simulink model "EVdemo_6"  (R2013b)
settings: Solver=FixedStepDiscrete  SolverMode=SingleTasking  StartTime=0.0  StopTime=650  FixedStep=4e-5  MaxStep=1e-5  RelTol=1e-3
InitFcn:
  | %EV_Param_Update
  | % update the number of strings (discretized)
  | numStrings = round(Opti_numStrings);
  | %disp(['Number of strings: ' num2str(numStrings)])
  | % update the effective capacity based on the number of strings
  | EV_Param.Battery_Det.Rated_Capacity = 28.5*numStrings; %A*hr
  | EV_Param.Battery_Det.DP = 1.5*fliplr([1500 1500 1600 1450 1325 1125 925 675 425 175 ])./8*EV_Param.Battery_Det.Rated_Capacity; % 8 comes from the 8Ahr rated batter data used (normalize and rescale to the rated capacity
  | EV_Param.Battery_Det.CP = fliplr([25 100 200 250 375 550 750 950 1125 1150])./8*EV_Param.Battery_Det.Rated_Capacity;
  | 
  | % update the number of cells in a string (discretized)
  | numSeriesCells = round(Opti_numSeriesCells);
  | %disp(['Number of cells in a string: ' num2str(numSeriesCells)])
  | % update the nominal string volage and charge deficit
  | EV_Param.Battery_Det.Nominal_Voltage = numSeriesCells*cellVolts;
  | BatteryParams(1).Qe_init = 0;%EV_Param.Battery_Det.Rated_Capacity*(1-EV_Param.Battery_Det.Initial_SOC/100); %Ampere*hours
  | 
  | % update the total number of cells, battery pack mass and total vehicle
  | % mass
  | total_cells = numSeriesCells*numStrings;
  | %disp(['Total Number of cells: ' num2str(total_cells)])
  | EV_Param.BatteryMass = BatteryParams(1).cell_mass*total_cells;
  | %disp(['Total Battery Pack Mass: ' num2str(EV_Param.BatteryMass)])
  | EV_Param.Vehicle.Mass = 1300+EV_Param.BatteryMass;
  | 
  | % update the driveline gear ratio
  | EV_Param.Vehicle.Engine_Vehicle_Gear_Ratio = Opti_Vehicle_Gear_Ratio;
  | %disp(['Driveline gear ratio: ' num2str(Opti_Vehicle_Gear_Ratio)])
StartFcn:
  | %tic;
StopFcn:
  | %toc;
  | %disp([Final SOC: ' num2str(SOC_final)])
  | %disp([Final Vehicle Error: ' num2str(normed_SQE_final)])
model workspace (MAT data in the model file):
  MCOS : class17 (value not decoded)
  MCOS : class17 (value not decoded)
values from neighbouring files (symbols this model uses):
  Drive_Cycle_Num = 8    [startDemo.m]
undefined symbols (not defined in the file or in its folder): Acc_Cmd, BatteryParams, Brake_Set, cell_area, ctrlConst, current_phase_a, Dec_Cmd, direct_current, DiscIntNeverNeededParam, electromagnetic_torque, HEV_Param, Ion, Kt_Temps, Lithium, Mech_Power_kW, Opti_numSeriesCells, Opti_numStrings, Opti_Vehicle_Gear_Ratio, paramVelocityI, paramVelocityP, paramVelocityPICurrentSat, pmsm, quadrature_current, RLoadLoss, rotor_velocity, sigbuilder_block, Ts, Veh_Spd_Ref
libraries: fl_lib x306, nesl_utility x100, LeadAcidBattery_lib x60, simulink x23, powerlib x16, sdl_lib x7, elec_lib x4, electricdrivelib x2, checkpacklib x2, CustomDriveline_lib x2, LiBatteryBlocks x1, Capacitors_lib x1
(part 4 of 7)

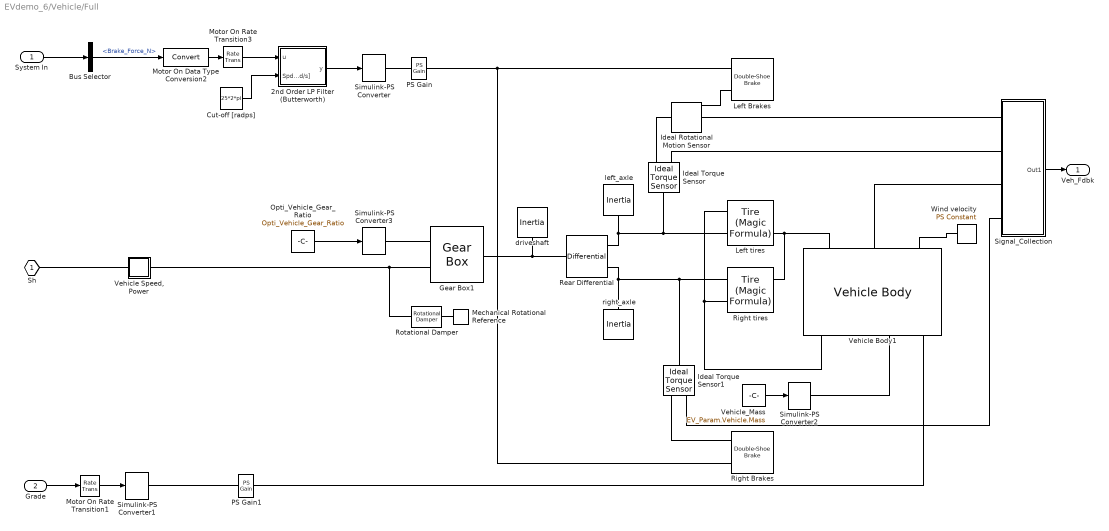
== system EVdemo_6/Vehicle/Full ==
  System In : Inport
  Grade : Inport  Port=2
  2nd Order LP Filter (Butterworth) : Subsystem  mask{DT=1e-3}
      mask prompts: DT "Sampe Time"
      mask Display:
      | plot([0 0],[0 1]);
      | plot([0 1],[0 0]);
      | plot([0 .5 .75 1],[1 1 .7071 .01]);
  Bus Selector : BusSelector  OutputSignals=Brake_Force_N
  Cut-off [radps] : Constant  Value=25*2*pi  OutDataTypeStr=single  SampleTime=-1
  Gear Box1 : CustomDriveline_lib/Gear Box  ratio_min=1  t_in_Log=off  t_out_Log=off  LocalVarNames=|t_in|t_out  LocalVarDescs=|t_in|t_out  LocalVarLogging=[0 0]
  Ideal Rotational Motion Sensor : fl_lib/Mechanical/Mechanical Sensors/Ideal Rotational Motion Sensor  offset=0 rad  w_Log=off  t_Log=off  phi_Log=off  LocalVarNames=|w|t|phi  LocalVarDescs=|w|t|phi  LocalVarLogging=[0 0 0]
  Ideal Torque Sensor : fl_lib/Mechanical/Mechanical Sensors/Ideal Torque Sensor  w_Log=off  t_Log=off  LocalVarNames=|w|t  LocalVarDescs=|w|t  LocalVarLogging=[0 0]
  Ideal Torque Sensor1 : fl_lib/Mechanical/Mechanical Sensors/Ideal Torque Sensor  w_Log=off  t_Log=off  LocalVarNames=|w|t  LocalVarDescs=|w|t  LocalVarLogging=[0 0]
  Left Brakes : sdl_lib/Brakes & Detents/Rotational/Double-Shoe Brake  r_drum=150 mm  r_act=125 mm  r_pin=125 mm  theta_pin=15 deg  theta_0=5 deg  theta_shoe=120 deg  mu_visc=.01 N*m/(rad/s)  mu=0.3  w_thr=0.1 rad/s  w_shaft_Log=off  t_shaft_Log=off  LocalVarNames=|w_shaft|t_shaft  LocalVarDescs=|Rotational velocity of the shaft|Braking torque on the shaft  LocalVarLogging=[0 0]  mask(Double-Shoe Brake){}
      mask Display:
      | % This is a new mask on top of the base mask.
      | % Use "View base mask" link below to see the base mask.
      | image('brakes.jpg')
  Left tires : sdl_lib/Tires & Vehicles/Tire (Magic Formula)  parameterization=1  F_z1=EV_Param.Vehicle.Tire.Rated_Vertical_Load N  F_x1=EV_Param.Vehicle.Tire.Rated_Peak_Long_Force N  kappa1=EV_Param.Vehicle.Tire.Slip_At_Peak_Force  B_m=10  C_m=1.9  D_m=1  E_m=0.97  fz0=4e+3 N  p_Cx=1.685  p_Dx=[ 1.21 -0.037 ]  p_Ex=[ 0.344 0.095 -0.02 0 ]  p_Kx=[ 21.51 -0.163 0.245 ]  p_Hx=[ -0.002 0.002 ]  p_Vx=[ 0 0 ]  v_tr_thr=0.1 m/s  r_e=EV_Param.Vehicle.Tire_Radius m  model_compliance=0  stiffness=1e+6 N/m  damping=1000 N/(m/s)  model_inertia=1  inertia=1e-2 kg*m^2  initial_velocity=0 rpm  model_resistance=1  resistance_model=2  coeff=0.015  p_tire=250e3 Pa  alpha=-0.003  beta=0.97  coeff_a=84e-4  coeff_b=6.2e-4 s/m  coeff_c=1.6e-4 s^2/m^2  v_thr=1e-2 m/s  LocalVarLogging=[]
  Mechanical Rotational Reference : fl_lib/Mechanical/Rotational Elements/Mechanical Rotational Reference  t_Log=off  LocalVarNames=|t  LocalVarDescs=|t  LocalVarLogging=0
  Motor On Data Type Conversion2 : DataTypeConversion
  Motor On Rate Transition1 : RateTransition  Deterministic=off
  Motor On Rate Transition3 : RateTransition  Deterministic=off
  Opti_Vehicle_Gear_Ratio : Constant  Value=Opti_Vehicle_Gear_Ratio  OutDataTypeStr=double  SampleTime=-1
  PS Gain : fl_lib/Physical Signals/Functions/PS Gain  gain=1  LocalVarLogging=[]
  PS Gain1 : fl_lib/Physical Signals/Functions/PS Gain  gain=1  LocalVarLogging=[]
  Rear Differential : sdl_lib/Gears/Differential  driveshaft_location=2  cd_ratio=1  friction_model=1  efficiency=[ 0.85 0.92 ]  mu_visc=[ 0 0 ] N*m/(rad/s)  w_thr=[ 0.01 0.01 ] rad/s  LocalVarLogging=[]
  Right Brakes : sdl_lib/Brakes & Detents/Rotational/Double-Shoe Brake  r_drum=150 mm  r_act=125 mm  r_pin=125 mm  theta_pin=15 deg  theta_0=5 deg  theta_shoe=120 deg  mu_visc=.01 N*m/(rad/s)  mu=0.3  w_thr=0.1 rad/s  w_shaft_Log=off  t_shaft_Log=off  LocalVarNames=|w_shaft|t_shaft  LocalVarDescs=|Rotational velocity of the shaft|Braking torque on the shaft  LocalVarLogging=[0 0]  mask(Double-Shoe Brake){}
      mask Display:
      | % This is a new mask on top of the base mask.
      | % Use "View base mask" link below to see the base mask.
      | image('brakes.jpg')
  Right tires : sdl_lib/Tires & Vehicles/Tire (Magic Formula)  parameterization=1  F_z1=EV_Param.Vehicle.Tire.Rated_Vertical_Load N  F_x1=EV_Param.Vehicle.Tire.Rated_Peak_Long_Force N  kappa1=EV_Param.Vehicle.Tire.Slip_At_Peak_Force  B_m=10  C_m=1.9  D_m=1  E_m=0.97  fz0=4e+3 N  p_Cx=1.685  p_Dx=[ 1.21 -0.037 ]  p_Ex=[ 0.344 0.095 -0.02 0 ]  p_Kx=[ 21.51 -0.163 0.245 ]  p_Hx=[ -0.002 0.002 ]  p_Vx=[ 0 0 ]  v_tr_thr=0.1 m/s  r_e=EV_Param.Vehicle.Tire_Radius m  model_compliance=0  stiffness=1e+6 N/m  damping=1000 N/(m/s)  model_inertia=1  inertia=1e-2 kg*m^2  initial_velocity=0 rpm  model_resistance=1  resistance_model=2  coeff=0.015  p_tire=250e3 Pa  alpha=-0.003  beta=0.97  coeff_a=84e-4  coeff_b=6.2e-4 s/m  coeff_c=1.6e-4 s^2/m^2  v_thr=1e-2 m/s  LocalVarLogging=[]
  Rotational Damper : fl_lib/Mechanical/Rotational Elements/Rotational Damper  D=EV_Param.Vehicle.Trans.Friction N*m/(rad/s)  t_Log=off  w_Log=off  LocalVarNames=|t|w  LocalVarDescs=|t|w  LocalVarLogging=[0 0]
  Signal_Collection : Subsystem
  Simulink-PS Converter : nesl_utility/Simulink-PS Converter  PhysicalDomain=network_engine_domain  SubClassName=ps_input  LeftPortType=input  RightPortType=output  PseudoPeriodic=off  Frequencies=[]  NoiseDistribution=none  NoiseParameters=[]  Unit=N  AffineConversion=off  InputFiltering=off  SimscapeFilterOrder=1  InputFilterTimeConstant=0.001  UdotUserProvided=1
  Simulink-PS Converter1 : nesl_utility/Simulink-PS Converter  PhysicalDomain=network_engine_domain  SubClassName=ps_input  LeftPortType=input  RightPortType=output  PseudoPeriodic=off  Frequencies=[]  NoiseDistribution=none  NoiseParameters=[]  Unit=rad  AffineConversion=off  InputFiltering=off  SimscapeFilterOrder=1  InputFilterTimeConstant=0.001  UdotUserProvided=1
  Simulink-PS Converter2 : nesl_utility/Simulink-PS Converter  PhysicalDomain=network_engine_domain  SubClassName=ps_input  LeftPortType=input  RightPortType=output  PseudoPeriodic=off  Frequencies=[]  NoiseDistribution=none  NoiseParameters=[]  Unit=kg  AffineConversion=off  InputFiltering=off  SimscapeFilterOrder=1  InputFilterTimeConstant=0.001  UdotUserProvided=1
  Simulink-PS Converter3 : nesl_utility/Simulink-PS Converter  PhysicalDomain=network_engine_domain  SubClassName=ps_input  LeftPortType=input  RightPortType=output  PseudoPeriodic=off  Frequencies=[]  NoiseDistribution=none  NoiseParameters=[]  Unit=1  AffineConversion=off  InputFiltering=off  SimscapeFilterOrder=1  InputFilterTimeConstant=0.001  UdotUserProvided=1
  "Vehicle Speed, Power" : Subsystem
      mask Display: disp('S')
  Vehicle Body1 : CustomDriveline_lib/Vehicle Body  n_w=2  x_f=EV_Param.Vehicle.Distance_CG_FrontAxle m  x_r=EV_Param.Vehicle.Distance_CG_RearAxle m  y_c=EV_Param.Vehicle.Distance_CG_Ground m  area=EV_Param.Vehicle.Frontal_Area m^2  Cd=EV_Param.Vehicle.Aero_Drag_Coeff  v0=0 m/s  g=9.81 m/s^2  rho=1.18 kg/m^3  mass_min=1e-3 kg  LocalVarLogging=[]
  Vehicle_Mass : Constant  Value=EV_Param.Vehicle.Mass  OutDataTypeStr=double  SampleTime=-1
  Wind velocity : fl_lib/Physical Signals/Sources/PS Constant  constant=0  LocalVarLogging=[]
  driveshaft : fl_lib/Mechanical/Rotational Elements/Inertia  inertia=EV_Param.Vehicle.Trans.Inertia kg*m^2  initial_velocity=0 rad/s  t_Log=off  LocalVarNames=|t  LocalVarDescs=|t  LocalVarLogging=0
  left_axle : fl_lib/Mechanical/Rotational Elements/Inertia  inertia=EV_Param.Vehicle.Wheel_Inertia*2 kg*m^2  initial_velocity=0 rad/s  t_Log=off  LocalVarNames=|t  LocalVarDescs=|t  LocalVarLogging=0
  right_axle : fl_lib/Mechanical/Rotational Elements/Inertia  inertia=EV_Param.Vehicle.Wheel_Inertia*2 kg*m^2  initial_velocity=0 rad/s  t_Log=off  LocalVarNames=|t  LocalVarDescs=|t  LocalVarLogging=0
  Sh : PMIOPort  Port=1  Side=Left
  Veh_Fdbk : Outport
  wires:
  Bus Selector/1 -> Motor On Data Type Conversion2/1  "<Brake_Force_N>"
  System In/1 -> Bus Selector/1
  Motor On Data Type Conversion2/1 -> Motor On Rate Transition3/1
  Motor On Rate Transition1/1 -> Simulink-PS Converter1/1
  Grade/1 -> Motor On Rate Transition1/1
  Signal_Collection/1(Out1) -> Veh_Fdbk/1
  Motor On Rate Transition3/1 -> 2nd Order LP Filter (Butterworth)/1(u)
  Cut-off [radps]/1 -> 2nd Order LP Filter (Butterworth)/2(Spd_Err_Filt_BW [rad/s])
  2nd Order LP Filter (Butterworth)/1(y) -> Simulink-PS Converter/1
  Vehicle_Mass/1 -> Simulink-PS Converter2/1
  Opti_Vehicle_Gear_Ratio/1 -> Simulink-PS Converter3/1
  connections:
  Right tires/RConn2 -- Vehicle Body1/LConn1 -- Left tires/RConn2
  Right tires/LConn1 -- Left tires/LConn1 -- Vehicle Body1/RConn1
  PS Gain1/RConn1 -- Vehicle Body1/RConn4
  Wind velocity/RConn1 -- Vehicle Body1/LConn3
  Rear Differential/RConn2 -- Left tires/LConn2 -- Ideal Torque Sensor/LConn1 -- left_axle/LConn1
  Right tires/LConn2 -- Ideal Torque Sensor1/LConn1 -- Rear Differential/RConn1 -- right_axle/LConn1
  Rear Differential/LConn1 -- Gear Box1/RConn1 -- driveshaft/LConn1
  "Vehicle Speed, Power"/RConn1 -- Gear Box1/LConn2 -- Rotational Damper/LConn1
  Rotational Damper/RConn1 -- Mechanical Rotational Reference/LConn1
  Sh/RConn1 -- "Vehicle Speed, Power"/LConn1
  PS Gain/RConn1 -- Right Brakes/LConn1 -- Left Brakes/LConn1
  Simulink-PS Converter/RConn1 -- PS Gain/LConn1
  Simulink-PS Converter1/RConn1 -- PS Gain1/LConn1
  Ideal Torque Sensor/RConn1 -- Ideal Rotational Motion Sensor/LConn1
  Ideal Torque Sensor1/RConn1 -- Right Brakes/LConn2
  Ideal Rotational Motion Sensor/RConn1 -- Left Brakes/LConn2
  Ideal Rotational Motion Sensor/RConn2 -- Signal_Collection/LConn1
  Ideal Torque Sensor/RConn2 -- Signal_Collection/LConn2
  Vehicle Body1/LConn2 -- Signal_Collection/LConn3
  Ideal Torque Sensor1/RConn2 -- Signal_Collection/LConn4
  Simulink-PS Converter2/RConn1 -- Vehicle Body1/RConn3
  Simulink-PS Converter3/RConn1 -- Gear Box1/LConn1

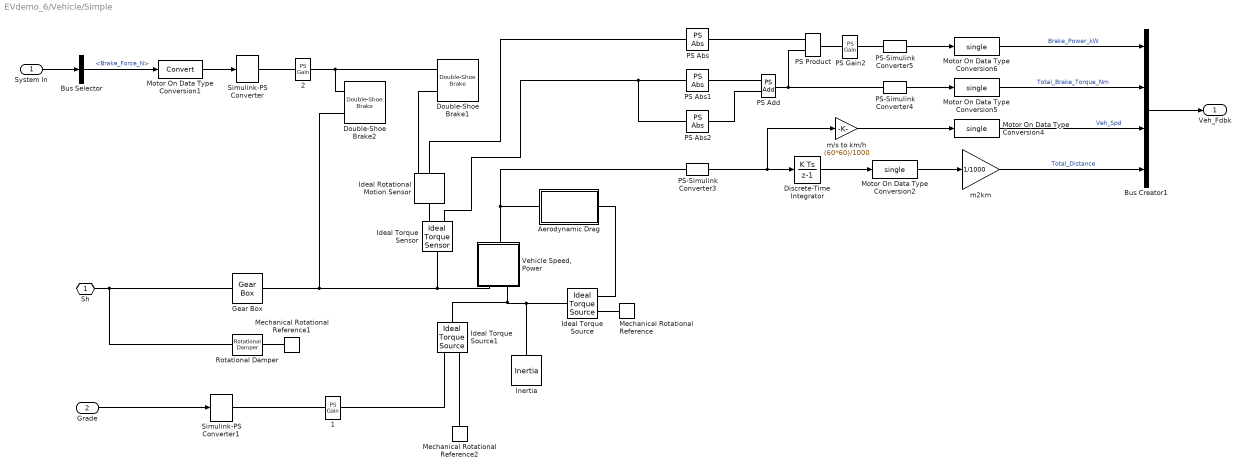
== system EVdemo_6/Vehicle/Simple ==
  System In : Inport
  Grade : Inport  Port=2
  1 : fl_lib/Physical Signals/Functions/PS Gain  gain=0  LocalVarLogging=[]
  2 : fl_lib/Physical Signals/Functions/PS Gain  gain=1  LocalVarLogging=[]
  Aerodynamic Drag : Subsystem
  Bus Creator1 : BusCreator
  Bus Selector : BusSelector  OutputSignals=Brake_Force_N
  Discrete-Time Integrator : DiscreteIntegrator  SampleTime=-1  ICPrevOutput=DiscIntNeverNeededParam  ICPrevScaledInput=DiscIntNeverNeededParam
  Double-Shoe Brake1 : sdl_lib/Brakes & Detents/Rotational/Double-Shoe Brake  r_drum=150 mm  r_act=125 mm  r_pin=125 mm  theta_pin=15 deg  theta_0=5 deg  theta_shoe=120 deg  mu_visc=.01 N*m/(rad/s)  mu=0.3  w_thr=0.1 rad/s  w_shaft_Log=off  t_shaft_Log=off  LocalVarNames=|w_shaft|t_shaft  LocalVarDescs=|Rotational velocity of the shaft|Braking torque on the shaft  LocalVarLogging=[0 0]
  Double-Shoe Brake2 : sdl_lib/Brakes & Detents/Rotational/Double-Shoe Brake  r_drum=150 mm  r_act=125 mm  r_pin=125 mm  theta_pin=15 deg  theta_0=5 deg  theta_shoe=120 deg  mu_visc=.01 N*m/(rad/s)  mu=0.3  w_thr=0.1 rad/s  w_shaft_Log=off  t_shaft_Log=off  LocalVarNames=|w_shaft|t_shaft  LocalVarDescs=|Rotational velocity of the shaft|Braking torque on the shaft  LocalVarLogging=[0 0]
  Gear Box : fl_lib/Mechanical/Mechanisms/Gear Box  ratio=gear_ratio  t_in_Log=off  t_out_Log=off  LocalVarNames=|t_in|t_out  LocalVarDescs=|t_in|t_out  LocalVarLogging=[0 0]
  Ideal Rotational Motion Sensor : fl_lib/Mechanical/Mechanical Sensors/Ideal Rotational Motion Sensor  offset=0 rad  w_Log=off  t_Log=off  phi_Log=off  LocalVarNames=|w|t|phi  LocalVarDescs=|w|t|phi  LocalVarLogging=[0 0 0]
  Ideal Torque Sensor : fl_lib/Mechanical/Mechanical Sensors/Ideal Torque Sensor  w_Log=off  t_Log=off  LocalVarNames=|w|t  LocalVarDescs=|w|t  LocalVarLogging=[0 0]
  Ideal Torque Source : fl_lib/Mechanical/Mechanical Sources/Ideal Torque Source  w_Log=off  t_Log=off  LocalVarNames=|w|t  LocalVarDescs=|w|t  LocalVarLogging=[0 0]
  Ideal Torque Source1 : fl_lib/Mechanical/Mechanical Sources/Ideal Torque Source  w_Log=off  t_Log=off  LocalVarNames=|w|t  LocalVarDescs=|w|t  LocalVarLogging=[0 0]
  Inertia : fl_lib/Mechanical/Rotational Elements/Inertia  inertia=4*wheel_inertia+mass*radius*radius kg*m^2  initial_velocity=0 rad/s  t_Log=off  LocalVarNames=|t  LocalVarDescs=|t  LocalVarLogging=0
  Mechanical Rotational Reference : fl_lib/Mechanical/Rotational Elements/Mechanical Rotational Reference  t_Log=off  LocalVarNames=|t  LocalVarDescs=|t  LocalVarLogging=0
  Mechanical Rotational Reference1 : fl_lib/Mechanical/Rotational Elements/Mechanical Rotational Reference  t_Log=off  LocalVarNames=|t  LocalVarDescs=|t  LocalVarLogging=0
  Mechanical Rotational Reference2 : fl_lib/Mechanical/Rotational Elements/Mechanical Rotational Reference  t_Log=off  LocalVarNames=|t  LocalVarDescs=|t  LocalVarLogging=0
  Motor On Data Type Conversion1 : DataTypeConversion
  Motor On Data Type Conversion{2,4..6} (4 alike) : DataTypeConversion  OutDataTypeStr=single
  PS Abs : fl_lib/Physical Signals/Nonlinear Operators/PS Abs  LocalVarLogging=[]
  PS Abs1 : fl_lib/Physical Signals/Nonlinear Operators/PS Abs  LocalVarLogging=[]
  PS Abs2 : fl_lib/Physical Signals/Nonlinear Operators/PS Abs  LocalVarLogging=[]
  PS Add : fl_lib/Physical Signals/Functions/PS Add  LocalVarLogging=[]
  PS Gain2 : fl_lib/Physical Signals/Functions/PS Gain  gain=1e-3  LocalVarLogging=[]
  PS Product : fl_lib/Physical Signals/Functions/PS Product  LocalVarLogging=[]
  PS-Simulink Converter3 : nesl_utility/PS-Simulink Converter  PhysicalDomain=network_engine_domain  SubClassName=ps_output  LeftPortType=input  RightPortType=output  PseudoPeriodic=off  Frequencies=[]  Unit=m/s  AffineConversion=off
  PS-Simulink Converter4 : nesl_utility/PS-Simulink Converter  PhysicalDomain=network_engine_domain  SubClassName=ps_output  LeftPortType=input  RightPortType=output  PseudoPeriodic=off  Frequencies=[]  Unit=m/s  AffineConversion=off
  PS-Simulink Converter5 : nesl_utility/PS-Simulink Converter  PhysicalDomain=network_engine_domain  SubClassName=ps_output  LeftPortType=input  RightPortType=output  PseudoPeriodic=off  Frequencies=[]  Unit=m/s  AffineConversion=off
  Rotational Damper : fl_lib/Mechanical/Rotational Elements/Rotational Damper  D=EV_Param.Vehicle.Trans.Friction N*m/(rad/s)  t_Log=off  w_Log=off  LocalVarNames=|t|w  LocalVarDescs=|t|w  LocalVarLogging=[0 0]
  Simulink-PS Converter : nesl_utility/Simulink-PS Converter  PhysicalDomain=network_engine_domain  SubClassName=ps_input  LeftPortType=input  RightPortType=output  PseudoPeriodic=off  Frequencies=[]  NoiseDistribution=none  NoiseParameters=[]  Unit=N  AffineConversion=off  InputFiltering=off  SimscapeFilterOrder=1  InputFilterTimeConstant=0.001  UdotUserProvided=1
  Simulink-PS Converter1 : nesl_utility/Simulink-PS Converter  PhysicalDomain=network_engine_domain  SubClassName=ps_input  LeftPortType=input  RightPortType=output  PseudoPeriodic=off  Frequencies=[]  NoiseDistribution=none  NoiseParameters=[]  Unit=N  AffineConversion=off  InputFiltering=off  SimscapeFilterOrder=1  InputFilterTimeConstant=0.001  UdotUserProvided=1
  "Vehicle Speed, Power" : Subsystem
  m/s to km/h : Gain  Gain=(60*60)/1000
  m2km : Gain  Gain=1/1000
  Sh : PMIOPort  Port=1  Side=Left
  Veh_Fdbk : Outport
  wires:
  System In/1 -> Bus Selector/1
  Bus Selector/1 -> Motor On Data Type Conversion1/1  "<Brake_Force_N>"
  PS-Simulink Converter3/1 -> Discrete-Time Integrator/1, m/s to km/h/1
  Motor On Data Type Conversion4/1 -> Bus Creator1/3  "Veh_Spd"
  Motor On Data Type Conversion2/1 -> m2km/1
  Bus Creator1/1 -> Veh_Fdbk/1
  m2km/1 -> Bus Creator1/4  "Total_Distance"
  PS-Simulink Converter4/1 -> Motor On Data Type Conversion5/1
  PS-Simulink Converter5/1 -> Motor On Data Type Conversion6/1
  Motor On Data Type Conversion6/1 -> Bus Creator1/1  "Brake_Power_kW"
  Motor On Data Type Conversion5/1 -> Bus Creator1/2  "Total_Brake_Torque_Nm"
  m/s to km/h/1 -> Motor On Data Type Conversion4/1
  Discrete-Time Integrator/1 -> Motor On Data Type Conversion2/1
  Grade/1 -> Simulink-PS Converter1/1
  Motor On Data Type Conversion1/1 -> Simulink-PS Converter/1
  connections:
  Rotational Damper/LConn1 -- Sh/RConn1 -- Gear Box/LConn1
  "Vehicle Speed, Power"/RConn1 -- PS-Simulink Converter3/LConn1 -- Aerodynamic Drag/LConn1
  Ideal Torque Source/RConn1 -- Aerodynamic Drag/RConn1
  Mechanical Rotational Reference/LConn1 -- Ideal Torque Source/RConn2
  Ideal Torque Source/LConn1 -- Inertia/LConn1 -- Ideal Torque Source1/LConn1 -- "Vehicle Speed, Power"/LConn2
  Mechanical Rotational Reference1/LConn1 -- Rotational Damper/RConn1
  Gear Box/RConn1 -- Double-Shoe Brake2/LConn2 -- "Vehicle Speed, Power"/LConn1 -- Ideal Torque Sensor/LConn1
  2/RConn1 -- Double-Shoe Brake2/LConn1 -- Double-Shoe Brake1/LConn1
  Simulink-PS Converter/RConn1 -- 2/LConn1
  PS-Simulink Converter4/LConn1 -- PS Add/RConn1 -- PS Product/LConn2
  PS Product/RConn1 -- PS Gain2/LConn1
  PS Abs/RConn1 -- PS Product/LConn1
  PS Abs1/RConn1 -- PS Add/LConn1
  PS Abs2/RConn1 -- PS Add/LConn2
  PS Gain2/RConn1 -- PS-Simulink Converter5/LConn1
  Ideal Torque Sensor/RConn1 -- Ideal Rotational Motion Sensor/LConn1
  Ideal Rotational Motion Sensor/RConn1 -- Double-Shoe Brake1/LConn2
  Mechanical Rotational Reference2/LConn1 -- Ideal Torque Source1/RConn2
  1/RConn1 -- Ideal Torque Source1/RConn1
  Simulink-PS Converter1/RConn1 -- 1/LConn1
  Ideal Rotational Motion Sensor/RConn2 -- PS Abs/LConn1
  Ideal Torque Sensor/RConn2 -- PS Abs2/LConn1 -- PS Abs1/LConn1

== system EVdemo_6/Battery/Cells/Battery cell1 ==
  " DOC " : Subsystem
  " SOC " : Subsystem
  C1 : LeadAcidBattery_lib/Main Branch Capacitance, C1  Tau1=HEV_Param.Battery_Cell.Tau1 s  Cmin=1e-5 F  i_Log=off  Q_Log=off  LocalVarNames=|i|v|Q  LocalVarDescs=|Current through variable|Voltage across variable|Charge variable  LocalVarLogging=[0 0 0]
  Diode : fl_lib/Electrical/Electrical Elements/Diode  Vf=0.6 V  Ron=0.3 Ohm  Goff=1e-08 1/Ohm  i_Log=off  v_Log=off  LocalVarNames=|current|voltage|power  LocalVarDescs=|Diode current (A)|Voltage across diode (V)|Power (W)  LocalVarLogging=[0 0 0]
  Ep : fl_lib/Electrical/Electrical Sources/DC Voltage Source  v0=HEV_Param.Battery_Cell.Ep V  i_Log=off  v_Log=off  LocalVarNames=|current|voltage|power  LocalVarDescs=|Current (A)|Voltage (V)|Power (W)  LocalVarLogging=[0 0 0]
  Main Branch Voltage Source (Em) : LeadAcidBattery_lib/Main Branch Voltage Source, Em  Em0=HEV_Param.Battery_Cell.Emo V  Ke=HEV_Param.Battery_Cell.Ke V/K  Kc=HEV_Param.Battery_Cell.Kc  C0=HEV_Param.Battery_Cell.Costar s*A  Istar=HEV_Param.Battery_Cell.Istar A  delta=HEV_Param.Battery_Cell.delta  Tau1=HEV_Param.Battery_Cell.Tau1 s  Qinit=HEV_Param.Battery_Cell.Qe_init s*A  i_Log=off  Iavg_Log=off  Qe_Log=off  LocalVarNames=|i|v|cap_u|cap_t|Q|Iavg  LocalVarDescs=|Current through variable|Voltage across variable|usable battery capacity|total battery capacity|battery charge|average current given by (I/(Ts+1))  LocalVarLogging=[0 0 0 0 0 0]
  R0 : LeadAcidBattery_lib/Terminal Resistance, R0  R00=HEV_Param.Battery_Cell.Roo Ohm  A0=HEV_Param.Battery_Cell.Ao  i_Log=off  LocalVarNames=|i|v  LocalVarDescs=|Current through variable|Voltage across variable  LocalVarLogging=[0 0]
  R1 : LeadAcidBattery_lib/Main Branch Resistance, R1  R10=HEV_Param.Battery_Cell.R10 Ohm  DOC_min=1e-006  i_Log=off  LocalVarNames=|i|v  LocalVarDescs=|Current through variable|Voltage across variable  LocalVarLogging=[0 0]
  R2 : LeadAcidBattery_lib/Main Branch Resistance, R2  R20=HEV_Param.Battery_Cell.R20 Ohm  A21=HEV_Param.Battery_Cell.A21  A22=HEV_Param.Battery_Cell.A22  Istar=HEV_Param.Battery_Cell.Istar A  i_Log=off  LocalVarNames=|i|v  LocalVarDescs=|Current through variable|Voltage across variable  LocalVarLogging=[0 0]
  Rp : LeadAcidBattery_lib/Parasitic Branch Resistance, Rp  Gp0=HEV_Param.Battery_Cell.Gpo 1/Ohm  Vp0=HEV_Param.Battery_Cell.Vpo V  Ap=HEV_Param.Battery_Cell.Ap  Tf=HEV_Param.Battery_Cell.theta_f C  i_Log=off  LocalVarNames=|i|v|Vavg  LocalVarDescs=|Current through variable|Voltage across variable|average voltage given by (V/(Ts+1))  LocalVarLogging=[0 0 0]
  T : Subsystem
  Thermal Model : Subsystem
  H : PMIOPort  Tag=PMCPort  Port=1  Side=Left
  + : PMIOPort  Tag=PMCPort  Port=2  Side=Left
  - : PMIOPort  Tag=PMCPort  Port=3  Side=Right
  connections:
  Diode/LConn1 -- R0/RConn1 -- R2/LConn2
  R2/RConn2 -- Thermal Model/LConn1
  -/RConn1 -- Ep/RConn1 -- Main Branch Voltage Source (Em)/RConn1
  Thermal Model/RConn1 -- Main Branch Voltage Source (Em)/RConn3
  Diode/RConn1 -- Rp/LConn1
  Ep/LConn1 -- Rp/RConn2
  Thermal Model/LConn2 -- H/RConn1
  R2/LConn1 -- Main Branch Voltage Source (Em)/LConn1 -- R0/LConn1 -- " SOC "/LConn1
  R1/LConn2 -- C1/LConn1
  R1/LConn1 -- C1/LConn2 -- R2/RConn1
  Main Branch Voltage Source (Em)/LConn3 -- C1/RConn1 -- R1/RConn2
  Main Branch Voltage Source (Em)/LConn2 -- R1/RConn1 -- " DOC "/LConn1
  R0/LConn2 -- +/RConn1
  Main Branch Voltage Source (Em)/RConn2 -- Rp/RConn1 -- T/LConn1 -- Thermal Model/RConn2

== system EVdemo_6/Battery/Cells/Battery cell10 ==
  C1 : LeadAcidBattery_lib/Main Branch Capacitance, C1  Tau1=HEV_Param.Battery_Cell.Tau1 s  Cmin=1e-5 F  i_Log=off  Q_Log=off  LocalVarNames=|i|v|Q  LocalVarDescs=|Current through variable|Voltage across variable|Charge variable  LocalVarLogging=[0 0 0]
  Diode : fl_lib/Electrical/Electrical Elements/Diode  Vf=0.6 V  Ron=0.3 Ohm  Goff=1e-08 1/Ohm  i_Log=off  v_Log=off  LocalVarNames=|current|voltage|power  LocalVarDescs=|Diode current (A)|Voltage across diode (V)|Power (W)  LocalVarLogging=[0 0 0]
  Ep : fl_lib/Electrical/Electrical Sources/DC Voltage Source  v0=HEV_Param.Battery_Cell.Ep V  i_Log=off  v_Log=off  LocalVarNames=|current|voltage|power  LocalVarDescs=|Current (A)|Voltage (V)|Power (W)  LocalVarLogging=[0 0 0]
  Main Branch Voltage Source (Em) : LeadAcidBattery_lib/Main Branch Voltage Source, Em  Em0=HEV_Param.Battery_Cell.Emo V  Ke=HEV_Param.Battery_Cell.Ke V/K  Kc=HEV_Param.Battery_Cell.Kc  C0=HEV_Param.Battery_Cell.Costar s*A  Istar=HEV_Param.Battery_Cell.Istar A  delta=HEV_Param.Battery_Cell.delta  Tau1=HEV_Param.Battery_Cell.Tau1 s  Qinit=HEV_Param.Battery_Cell.Qe_init s*A  i_Log=off  Iavg_Log=off  Qe_Log=off  LocalVarNames=|i|v|cap_u|cap_t|Q|Iavg  LocalVarDescs=|Current through variable|Voltage across variable|usable battery capacity|total battery capacity|battery charge|average current given by (I/(Ts+1))  LocalVarLogging=[0 0 0 0 0 0]
  R0 : LeadAcidBattery_lib/Terminal Resistance, R0  R00=HEV_Param.Battery_Cell.Roo Ohm  A0=HEV_Param.Battery_Cell.Ao  i_Log=off  LocalVarNames=|i|v  LocalVarDescs=|Current through variable|Voltage across variable  LocalVarLogging=[0 0]
  R1 : LeadAcidBattery_lib/Main Branch Resistance, R1  R10=HEV_Param.Battery_Cell.R10 Ohm  DOC_min=1e-006  i_Log=off  LocalVarNames=|i|v  LocalVarDescs=|Current through variable|Voltage across variable  LocalVarLogging=[0 0]
  R2 : LeadAcidBattery_lib/Main Branch Resistance, R2  R20=HEV_Param.Battery_Cell.R20 Ohm  A21=HEV_Param.Battery_Cell.A21  A22=HEV_Param.Battery_Cell.A22  Istar=HEV_Param.Battery_Cell.Istar A  i_Log=off  LocalVarNames=|i|v  LocalVarDescs=|Current through variable|Voltage across variable  LocalVarLogging=[0 0]
  Rp : LeadAcidBattery_lib/Parasitic Branch Resistance, Rp  Gp0=HEV_Param.Battery_Cell.Gpo 1/Ohm  Vp0=HEV_Param.Battery_Cell.Vpo V  Ap=HEV_Param.Battery_Cell.Ap  Tf=HEV_Param.Battery_Cell.theta_f C  i_Log=off  LocalVarNames=|i|v|Vavg  LocalVarDescs=|Current through variable|Voltage across variable|average voltage given by (V/(Ts+1))  LocalVarLogging=[0 0 0]
  Thermal Model : Subsystem
  H : PMIOPort  Tag=PMCPort  Port=1  Side=Left
  + : PMIOPort  Tag=PMCPort  Port=2  Side=Left
  - : PMIOPort  Tag=PMCPort  Port=3  Side=Right
  connections:
  Diode/LConn1 -- R0/RConn1 -- R2/LConn2
  R2/RConn2 -- Thermal Model/LConn1
  -/RConn1 -- Ep/RConn1 -- Main Branch Voltage Source (Em)/RConn1
  Thermal Model/RConn1 -- Main Branch Voltage Source (Em)/RConn3
  Diode/RConn1 -- Rp/LConn1
  Ep/LConn1 -- Rp/RConn2
  Thermal Model/LConn2 -- H/RConn1
  R0/LConn1 -- R2/LConn1 -- Main Branch Voltage Source (Em)/LConn1
  R1/LConn2 -- C1/LConn1
  R1/LConn1 -- C1/LConn2 -- R2/RConn1
  Main Branch Voltage Source (Em)/LConn3 -- C1/RConn1 -- R1/RConn2
  R1/RConn1 -- Main Branch Voltage Source (Em)/LConn2
  R0/LConn2 -- +/RConn1
  Thermal Model/RConn2 -- Main Branch Voltage Source (Em)/RConn2 -- Rp/RConn1

== system EVdemo_6/Battery/Cells/Battery cell2 ==
  C1 : LeadAcidBattery_lib/Main Branch Capacitance, C1  Tau1=HEV_Param.Battery_Cell.Tau1 s  Cmin=1e-5 F  i_Log=off  Q_Log=off  LocalVarNames=|i|v|Q  LocalVarDescs=|Current through variable|Voltage across variable|Charge variable  LocalVarLogging=[0 0 0]
  Diode : fl_lib/Electrical/Electrical Elements/Diode  Vf=0.6 V  Ron=0.3 Ohm  Goff=1e-08 1/Ohm  i_Log=off  v_Log=off  LocalVarNames=|current|voltage|power  LocalVarDescs=|Diode current (A)|Voltage across diode (V)|Power (W)  LocalVarLogging=[0 0 0]
  Ep : fl_lib/Electrical/Electrical Sources/DC Voltage Source  v0=HEV_Param.Battery_Cell.Ep V  i_Log=off  v_Log=off  LocalVarNames=|current|voltage|power  LocalVarDescs=|Current (A)|Voltage (V)|Power (W)  LocalVarLogging=[0 0 0]
  Main Branch Voltage Source (Em) : LeadAcidBattery_lib/Main Branch Voltage Source, Em  Em0=HEV_Param.Battery_Cell.Emo V  Ke=HEV_Param.Battery_Cell.Ke V/K  Kc=HEV_Param.Battery_Cell.Kc  C0=HEV_Param.Battery_Cell.Costar s*A  Istar=HEV_Param.Battery_Cell.Istar A  delta=HEV_Param.Battery_Cell.delta  Tau1=HEV_Param.Battery_Cell.Tau1 s  Qinit=HEV_Param.Battery_Cell.Qe_init s*A  i_Log=off  Iavg_Log=off  Qe_Log=off  LocalVarNames=|i|v|cap_u|cap_t|Q|Iavg  LocalVarDescs=|Current through variable|Voltage across variable|usable battery capacity|total battery capacity|battery charge|average current given by (I/(Ts+1))  LocalVarLogging=[0 0 0 0 0 0]
  R0 : LeadAcidBattery_lib/Terminal Resistance, R0  R00=HEV_Param.Battery_Cell.Roo Ohm  A0=HEV_Param.Battery_Cell.Ao  i_Log=off  LocalVarNames=|i|v  LocalVarDescs=|Current through variable|Voltage across variable  LocalVarLogging=[0 0]
  R1 : LeadAcidBattery_lib/Main Branch Resistance, R1  R10=HEV_Param.Battery_Cell.R10 Ohm  DOC_min=1e-006  i_Log=off  LocalVarNames=|i|v  LocalVarDescs=|Current through variable|Voltage across variable  LocalVarLogging=[0 0]
  R2 : LeadAcidBattery_lib/Main Branch Resistance, R2  R20=HEV_Param.Battery_Cell.R20 Ohm  A21=HEV_Param.Battery_Cell.A21  A22=HEV_Param.Battery_Cell.A22  Istar=HEV_Param.Battery_Cell.Istar A  i_Log=off  LocalVarNames=|i|v  LocalVarDescs=|Current through variable|Voltage across variable  LocalVarLogging=[0 0]
  Rp : LeadAcidBattery_lib/Parasitic Branch Resistance, Rp  Gp0=HEV_Param.Battery_Cell.Gpo 1/Ohm  Vp0=HEV_Param.Battery_Cell.Vpo V  Ap=HEV_Param.Battery_Cell.Ap  Tf=HEV_Param.Battery_Cell.theta_f C  i_Log=off  LocalVarNames=|i|v|Vavg  LocalVarDescs=|Current through variable|Voltage across variable|average voltage given by (V/(Ts+1))  LocalVarLogging=[0 0 0]
  Thermal Model : Subsystem
  H : PMIOPort  Tag=PMCPort  Port=1  Side=Left
  + : PMIOPort  Tag=PMCPort  Port=2  Side=Left
  - : PMIOPort  Tag=PMCPort  Port=3  Side=Right
  connections:
  Rp/RConn1 -- Main Branch Voltage Source (Em)/RConn2 -- Thermal Model/RConn2
  R0/LConn2 -- +/RConn1
  R1/RConn1 -- Main Branch Voltage Source (Em)/LConn2
  R1/RConn2 -- C1/RConn1 -- Main Branch Voltage Source (Em)/LConn3
  R2/RConn1 -- C1/LConn2 -- R1/LConn1
  R1/LConn2 -- C1/LConn1
  Main Branch Voltage Source (Em)/LConn1 -- R2/LConn1 -- R0/LConn1
  Thermal Model/LConn2 -- H/RConn1
  Ep/LConn1 -- Rp/RConn2
  Diode/RConn1 -- Rp/LConn1
  Thermal Model/RConn1 -- Main Branch Voltage Source (Em)/RConn3
  Main Branch Voltage Source (Em)/RConn1 -- Ep/RConn1 -- -/RConn1
  R2/RConn2 -- Thermal Model/LConn1
  R2/LConn2 -- R0/RConn1 -- Diode/LConn1

== system EVdemo_6/Battery/Cells/Battery cell3 ==
  C1 : LeadAcidBattery_lib/Main Branch Capacitance, C1  Tau1=HEV_Param.Battery_Cell.Tau1 s  Cmin=1e-5 F  i_Log=off  Q_Log=off  LocalVarNames=|i|v|Q  LocalVarDescs=|Current through variable|Voltage across variable|Charge variable  LocalVarLogging=[0 0 0]
  Diode : fl_lib/Electrical/Electrical Elements/Diode  Vf=0.6 V  Ron=0.3 Ohm  Goff=1e-08 1/Ohm  i_Log=off  v_Log=off  LocalVarNames=|current|voltage|power  LocalVarDescs=|Diode current (A)|Voltage across diode (V)|Power (W)  LocalVarLogging=[0 0 0]
  Ep : fl_lib/Electrical/Electrical Sources/DC Voltage Source  v0=HEV_Param.Battery_Cell.Ep V  i_Log=off  v_Log=off  LocalVarNames=|current|voltage|power  LocalVarDescs=|Current (A)|Voltage (V)|Power (W)  LocalVarLogging=[0 0 0]
  Main Branch Voltage Source (Em) : LeadAcidBattery_lib/Main Branch Voltage Source, Em  Em0=HEV_Param.Battery_Cell.Emo V  Ke=HEV_Param.Battery_Cell.Ke V/K  Kc=HEV_Param.Battery_Cell.Kc  C0=HEV_Param.Battery_Cell.Costar s*A  Istar=HEV_Param.Battery_Cell.Istar A  delta=HEV_Param.Battery_Cell.delta  Tau1=HEV_Param.Battery_Cell.Tau1 s  Qinit=HEV_Param.Battery_Cell.Qe_init s*A  i_Log=off  Iavg_Log=off  Qe_Log=off  LocalVarNames=|i|v|cap_u|cap_t|Q|Iavg  LocalVarDescs=|Current through variable|Voltage across variable|usable battery capacity|total battery capacity|battery charge|average current given by (I/(Ts+1))  LocalVarLogging=[0 0 0 0 0 0]
  R0 : LeadAcidBattery_lib/Terminal Resistance, R0  R00=HEV_Param.Battery_Cell.Roo Ohm  A0=HEV_Param.Battery_Cell.Ao  i_Log=off  LocalVarNames=|i|v  LocalVarDescs=|Current through variable|Voltage across variable  LocalVarLogging=[0 0]
  R1 : LeadAcidBattery_lib/Main Branch Resistance, R1  R10=HEV_Param.Battery_Cell.R10 Ohm  DOC_min=1e-006  i_Log=off  LocalVarNames=|i|v  LocalVarDescs=|Current through variable|Voltage across variable  LocalVarLogging=[0 0]
  R2 : LeadAcidBattery_lib/Main Branch Resistance, R2  R20=HEV_Param.Battery_Cell.R20 Ohm  A21=HEV_Param.Battery_Cell.A21  A22=HEV_Param.Battery_Cell.A22  Istar=HEV_Param.Battery_Cell.Istar A  i_Log=off  LocalVarNames=|i|v  LocalVarDescs=|Current through variable|Voltage across variable  LocalVarLogging=[0 0]
  Rp : LeadAcidBattery_lib/Parasitic Branch Resistance, Rp  Gp0=HEV_Param.Battery_Cell.Gpo 1/Ohm  Vp0=HEV_Param.Battery_Cell.Vpo V  Ap=HEV_Param.Battery_Cell.Ap  Tf=HEV_Param.Battery_Cell.theta_f C  i_Log=off  LocalVarNames=|i|v|Vavg  LocalVarDescs=|Current through variable|Voltage across variable|average voltage given by (V/(Ts+1))  LocalVarLogging=[0 0 0]
  Thermal Model : Subsystem
  H : PMIOPort  Tag=PMCPort  Port=1  Side=Left
  + : PMIOPort  Tag=PMCPort  Port=2  Side=Left
  - : PMIOPort  Tag=PMCPort  Port=3  Side=Right
  connections:
  Diode/LConn1 -- R0/RConn1 -- R2/LConn2
  R2/RConn2 -- Thermal Model/LConn1
  -/RConn1 -- Ep/RConn1 -- Main Branch Voltage Source (Em)/RConn1
  Thermal Model/RConn1 -- Main Branch Voltage Source (Em)/RConn3
  Diode/RConn1 -- Rp/LConn1
  Ep/LConn1 -- Rp/RConn2
  Thermal Model/LConn2 -- H/RConn1
  R0/LConn1 -- R2/LConn1 -- Main Branch Voltage Source (Em)/LConn1
  R1/LConn2 -- C1/LConn1
  R1/LConn1 -- C1/LConn2 -- R2/RConn1
  Main Branch Voltage Source (Em)/LConn3 -- C1/RConn1 -- R1/RConn2
  R1/RConn1 -- Main Branch Voltage Source (Em)/LConn2
  R0/LConn2 -- +/RConn1
  Thermal Model/RConn2 -- Main Branch Voltage Source (Em)/RConn2 -- Rp/RConn1

== system EVdemo_6/Battery/Cells/Battery cell4 ==
  C1 : LeadAcidBattery_lib/Main Branch Capacitance, C1  Tau1=HEV_Param.Battery_Cell.Tau1 s  Cmin=1e-5 F  i_Log=off  Q_Log=off  LocalVarNames=|i|v|Q  LocalVarDescs=|Current through variable|Voltage across variable|Charge variable  LocalVarLogging=[0 0 0]
  Diode : fl_lib/Electrical/Electrical Elements/Diode  Vf=0.6 V  Ron=0.3 Ohm  Goff=1e-08 1/Ohm  i_Log=off  v_Log=off  LocalVarNames=|current|voltage|power  LocalVarDescs=|Diode current (A)|Voltage across diode (V)|Power (W)  LocalVarLogging=[0 0 0]
  Ep : fl_lib/Electrical/Electrical Sources/DC Voltage Source  v0=HEV_Param.Battery_Cell.Ep V  i_Log=off  v_Log=off  LocalVarNames=|current|voltage|power  LocalVarDescs=|Current (A)|Voltage (V)|Power (W)  LocalVarLogging=[0 0 0]
  Main Branch Voltage Source (Em) : LeadAcidBattery_lib/Main Branch Voltage Source, Em  Em0=HEV_Param.Battery_Cell.Emo V  Ke=HEV_Param.Battery_Cell.Ke V/K  Kc=HEV_Param.Battery_Cell.Kc  C0=HEV_Param.Battery_Cell.Costar s*A  Istar=HEV_Param.Battery_Cell.Istar A  delta=HEV_Param.Battery_Cell.delta  Tau1=HEV_Param.Battery_Cell.Tau1 s  Qinit=HEV_Param.Battery_Cell.Qe_init s*A  i_Log=off  Iavg_Log=off  Qe_Log=off  LocalVarNames=|i|v|cap_u|cap_t|Q|Iavg  LocalVarDescs=|Current through variable|Voltage across variable|usable battery capacity|total battery capacity|battery charge|average current given by (I/(Ts+1))  LocalVarLogging=[0 0 0 0 0 0]
  R0 : LeadAcidBattery_lib/Terminal Resistance, R0  R00=HEV_Param.Battery_Cell.Roo Ohm  A0=HEV_Param.Battery_Cell.Ao  i_Log=off  LocalVarNames=|i|v  LocalVarDescs=|Current through variable|Voltage across variable  LocalVarLogging=[0 0]
  R1 : LeadAcidBattery_lib/Main Branch Resistance, R1  R10=HEV_Param.Battery_Cell.R10 Ohm  DOC_min=1e-006  i_Log=off  LocalVarNames=|i|v  LocalVarDescs=|Current through variable|Voltage across variable  LocalVarLogging=[0 0]
  R2 : LeadAcidBattery_lib/Main Branch Resistance, R2  R20=HEV_Param.Battery_Cell.R20 Ohm  A21=HEV_Param.Battery_Cell.A21  A22=HEV_Param.Battery_Cell.A22  Istar=HEV_Param.Battery_Cell.Istar A  i_Log=off  LocalVarNames=|i|v  LocalVarDescs=|Current through variable|Voltage across variable  LocalVarLogging=[0 0]
  Rp : LeadAcidBattery_lib/Parasitic Branch Resistance, Rp  Gp0=HEV_Param.Battery_Cell.Gpo 1/Ohm  Vp0=HEV_Param.Battery_Cell.Vpo V  Ap=HEV_Param.Battery_Cell.Ap  Tf=HEV_Param.Battery_Cell.theta_f C  i_Log=off  LocalVarNames=|i|v|Vavg  LocalVarDescs=|Current through variable|Voltage across variable|average voltage given by (V/(Ts+1))  LocalVarLogging=[0 0 0]
  Thermal Model : Subsystem
  H : PMIOPort  Tag=PMCPort  Port=1  Side=Left
  + : PMIOPort  Tag=PMCPort  Port=2  Side=Left
  - : PMIOPort  Tag=PMCPort  Port=3  Side=Right
  connections:
  Diode/LConn1 -- R0/RConn1 -- R2/LConn2
  R2/RConn2 -- Thermal Model/LConn1
  -/RConn1 -- Ep/RConn1 -- Main Branch Voltage Source (Em)/RConn1
  Thermal Model/RConn1 -- Main Branch Voltage Source (Em)/RConn3
  Diode/RConn1 -- Rp/LConn1
  Ep/LConn1 -- Rp/RConn2
  Thermal Model/LConn2 -- H/RConn1
  R0/LConn1 -- R2/LConn1 -- Main Branch Voltage Source (Em)/LConn1
  R1/LConn2 -- C1/LConn1
  R1/LConn1 -- C1/LConn2 -- R2/RConn1
  Main Branch Voltage Source (Em)/LConn3 -- C1/RConn1 -- R1/RConn2
  R1/RConn1 -- Main Branch Voltage Source (Em)/LConn2
  R0/LConn2 -- +/RConn1
  Thermal Model/RConn2 -- Main Branch Voltage Source (Em)/RConn2 -- Rp/RConn1

== system EVdemo_6/Battery/Cells/Battery cell5 ==
  C1 : LeadAcidBattery_lib/Main Branch Capacitance, C1  Tau1=HEV_Param.Battery_Cell.Tau1 s  Cmin=1e-5 F  i_Log=off  Q_Log=off  LocalVarNames=|i|v|Q  LocalVarDescs=|Current through variable|Voltage across variable|Charge variable  LocalVarLogging=[0 0 0]
  Diode : fl_lib/Electrical/Electrical Elements/Diode  Vf=0.6 V  Ron=0.3 Ohm  Goff=1e-08 1/Ohm  i_Log=off  v_Log=off  LocalVarNames=|current|voltage|power  LocalVarDescs=|Diode current (A)|Voltage across diode (V)|Power (W)  LocalVarLogging=[0 0 0]
  Ep : fl_lib/Electrical/Electrical Sources/DC Voltage Source  v0=HEV_Param.Battery_Cell.Ep V  i_Log=off  v_Log=off  LocalVarNames=|current|voltage|power  LocalVarDescs=|Current (A)|Voltage (V)|Power (W)  LocalVarLogging=[0 0 0]
  Main Branch Voltage Source (Em) : LeadAcidBattery_lib/Main Branch Voltage Source, Em  Em0=HEV_Param.Battery_Cell.Emo V  Ke=HEV_Param.Battery_Cell.Ke V/K  Kc=HEV_Param.Battery_Cell.Kc  C0=HEV_Param.Battery_Cell.Costar s*A  Istar=HEV_Param.Battery_Cell.Istar A  delta=HEV_Param.Battery_Cell.delta  Tau1=HEV_Param.Battery_Cell.Tau1 s  Qinit=HEV_Param.Battery_Cell.Qe_init s*A  i_Log=off  Iavg_Log=off  Qe_Log=off  LocalVarNames=|i|v|cap_u|cap_t|Q|Iavg  LocalVarDescs=|Current through variable|Voltage across variable|usable battery capacity|total battery capacity|battery charge|average current given by (I/(Ts+1))  LocalVarLogging=[0 0 0 0 0 0]
  R0 : LeadAcidBattery_lib/Terminal Resistance, R0  R00=HEV_Param.Battery_Cell.Roo Ohm  A0=HEV_Param.Battery_Cell.Ao  i_Log=off  LocalVarNames=|i|v  LocalVarDescs=|Current through variable|Voltage across variable  LocalVarLogging=[0 0]
  R1 : LeadAcidBattery_lib/Main Branch Resistance, R1  R10=HEV_Param.Battery_Cell.R10 Ohm  DOC_min=1e-006  i_Log=off  LocalVarNames=|i|v  LocalVarDescs=|Current through variable|Voltage across variable  LocalVarLogging=[0 0]
  R2 : LeadAcidBattery_lib/Main Branch Resistance, R2  R20=HEV_Param.Battery_Cell.R20 Ohm  A21=HEV_Param.Battery_Cell.A21  A22=HEV_Param.Battery_Cell.A22  Istar=HEV_Param.Battery_Cell.Istar A  i_Log=off  LocalVarNames=|i|v  LocalVarDescs=|Current through variable|Voltage across variable  LocalVarLogging=[0 0]
  Rp : LeadAcidBattery_lib/Parasitic Branch Resistance, Rp  Gp0=HEV_Param.Battery_Cell.Gpo 1/Ohm  Vp0=HEV_Param.Battery_Cell.Vpo V  Ap=HEV_Param.Battery_Cell.Ap  Tf=HEV_Param.Battery_Cell.theta_f C  i_Log=off  LocalVarNames=|i|v|Vavg  LocalVarDescs=|Current through variable|Voltage across variable|average voltage given by (V/(Ts+1))  LocalVarLogging=[0 0 0]
  Thermal Model : Subsystem
  H : PMIOPort  Tag=PMCPort  Port=1  Side=Left
  + : PMIOPort  Tag=PMCPort  Port=2  Side=Left
  - : PMIOPort  Tag=PMCPort  Port=3  Side=Right
  connections:
  Diode/LConn1 -- R0/RConn1 -- R2/LConn2
  R2/RConn2 -- Thermal Model/LConn1
  -/RConn1 -- Ep/RConn1 -- Main Branch Voltage Source (Em)/RConn1
  Thermal Model/RConn1 -- Main Branch Voltage Source (Em)/RConn3
  Diode/RConn1 -- Rp/LConn1
  Ep/LConn1 -- Rp/RConn2
  Thermal Model/LConn2 -- H/RConn1
  R0/LConn1 -- R2/LConn1 -- Main Branch Voltage Source (Em)/LConn1
  R1/LConn2 -- C1/LConn1
  R1/LConn1 -- C1/LConn2 -- R2/RConn1
  Main Branch Voltage Source (Em)/LConn3 -- C1/RConn1 -- R1/RConn2
  R1/RConn1 -- Main Branch Voltage Source (Em)/LConn2
  R0/LConn2 -- +/RConn1
  Thermal Model/RConn2 -- Main Branch Voltage Source (Em)/RConn2 -- Rp/RConn1

== system EVdemo_6/Battery/Cells/Battery cell6 ==
  C1 : LeadAcidBattery_lib/Main Branch Capacitance, C1  Tau1=HEV_Param.Battery_Cell.Tau1 s  Cmin=1e-5 F  i_Log=off  Q_Log=off  LocalVarNames=|i|v|Q  LocalVarDescs=|Current through variable|Voltage across variable|Charge variable  LocalVarLogging=[0 0 0]
  Diode : fl_lib/Electrical/Electrical Elements/Diode  Vf=0.6 V  Ron=0.3 Ohm  Goff=1e-08 1/Ohm  i_Log=off  v_Log=off  LocalVarNames=|current|voltage|power  LocalVarDescs=|Diode current (A)|Voltage across diode (V)|Power (W)  LocalVarLogging=[0 0 0]
  Ep : fl_lib/Electrical/Electrical Sources/DC Voltage Source  v0=HEV_Param.Battery_Cell.Ep V  i_Log=off  v_Log=off  LocalVarNames=|current|voltage|power  LocalVarDescs=|Current (A)|Voltage (V)|Power (W)  LocalVarLogging=[0 0 0]
  Main Branch Voltage Source (Em) : LeadAcidBattery_lib/Main Branch Voltage Source, Em  Em0=HEV_Param.Battery_Cell.Emo V  Ke=HEV_Param.Battery_Cell.Ke V/K  Kc=HEV_Param.Battery_Cell.Kc  C0=HEV_Param.Battery_Cell.Costar s*A  Istar=HEV_Param.Battery_Cell.Istar A  delta=HEV_Param.Battery_Cell.delta  Tau1=HEV_Param.Battery_Cell.Tau1 s  Qinit=HEV_Param.Battery_Cell.Qe_init s*A  i_Log=off  Iavg_Log=off  Qe_Log=off  LocalVarNames=|i|v|cap_u|cap_t|Q|Iavg  LocalVarDescs=|Current through variable|Voltage across variable|usable battery capacity|total battery capacity|battery charge|average current given by (I/(Ts+1))  LocalVarLogging=[0 0 0 0 0 0]
  R0 : LeadAcidBattery_lib/Terminal Resistance, R0  R00=HEV_Param.Battery_Cell.Roo Ohm  A0=HEV_Param.Battery_Cell.Ao  i_Log=off  LocalVarNames=|i|v  LocalVarDescs=|Current through variable|Voltage across variable  LocalVarLogging=[0 0]
  R1 : LeadAcidBattery_lib/Main Branch Resistance, R1  R10=HEV_Param.Battery_Cell.R10 Ohm  DOC_min=1e-006  i_Log=off  LocalVarNames=|i|v  LocalVarDescs=|Current through variable|Voltage across variable  LocalVarLogging=[0 0]
  R2 : LeadAcidBattery_lib/Main Branch Resistance, R2  R20=HEV_Param.Battery_Cell.R20 Ohm  A21=HEV_Param.Battery_Cell.A21  A22=HEV_Param.Battery_Cell.A22  Istar=HEV_Param.Battery_Cell.Istar A  i_Log=off  LocalVarNames=|i|v  LocalVarDescs=|Current through variable|Voltage across variable  LocalVarLogging=[0 0]
  Rp : LeadAcidBattery_lib/Parasitic Branch Resistance, Rp  Gp0=HEV_Param.Battery_Cell.Gpo 1/Ohm  Vp0=HEV_Param.Battery_Cell.Vpo V  Ap=HEV_Param.Battery_Cell.Ap  Tf=HEV_Param.Battery_Cell.theta_f C  i_Log=off  LocalVarNames=|i|v|Vavg  LocalVarDescs=|Current through variable|Voltage across variable|average voltage given by (V/(Ts+1))  LocalVarLogging=[0 0 0]
  Thermal Model : Subsystem
  H : PMIOPort  Tag=PMCPort  Port=1  Side=Left
  + : PMIOPort  Tag=PMCPort  Port=2  Side=Left
  - : PMIOPort  Tag=PMCPort  Port=3  Side=Right
  connections:
  Diode/LConn1 -- R0/RConn1 -- R2/LConn2
  R2/RConn2 -- Thermal Model/LConn1
  -/RConn1 -- Ep/RConn1 -- Main Branch Voltage Source (Em)/RConn1
  Thermal Model/RConn1 -- Main Branch Voltage Source (Em)/RConn3
  Diode/RConn1 -- Rp/LConn1
  Ep/LConn1 -- Rp/RConn2
  Thermal Model/LConn2 -- H/RConn1
  R0/LConn1 -- R2/LConn1 -- Main Branch Voltage Source (Em)/LConn1
  R1/LConn2 -- C1/LConn1
  R1/LConn1 -- C1/LConn2 -- R2/RConn1
  Main Branch Voltage Source (Em)/LConn3 -- C1/RConn1 -- R1/RConn2
  R1/RConn1 -- Main Branch Voltage Source (Em)/LConn2
  R0/LConn2 -- +/RConn1
  Thermal Model/RConn2 -- Main Branch Voltage Source (Em)/RConn2 -- Rp/RConn1

== system EVdemo_6/Battery/Cells/Battery cell7 ==
  C1 : LeadAcidBattery_lib/Main Branch Capacitance, C1  Tau1=HEV_Param.Battery_Cell.Tau1 s  Cmin=1e-5 F  i_Log=off  Q_Log=off  LocalVarNames=|i|v|Q  LocalVarDescs=|Current through variable|Voltage across variable|Charge variable  LocalVarLogging=[0 0 0]
  Diode : fl_lib/Electrical/Electrical Elements/Diode  Vf=0.6 V  Ron=0.3 Ohm  Goff=1e-08 1/Ohm  i_Log=off  v_Log=off  LocalVarNames=|current|voltage|power  LocalVarDescs=|Diode current (A)|Voltage across diode (V)|Power (W)  LocalVarLogging=[0 0 0]
  Ep : fl_lib/Electrical/Electrical Sources/DC Voltage Source  v0=HEV_Param.Battery_Cell.Ep V  i_Log=off  v_Log=off  LocalVarNames=|current|voltage|power  LocalVarDescs=|Current (A)|Voltage (V)|Power (W)  LocalVarLogging=[0 0 0]
  Main Branch Voltage Source (Em) : LeadAcidBattery_lib/Main Branch Voltage Source, Em  Em0=HEV_Param.Battery_Cell.Emo V  Ke=HEV_Param.Battery_Cell.Ke V/K  Kc=HEV_Param.Battery_Cell.Kc  C0=HEV_Param.Battery_Cell.Costar s*A  Istar=HEV_Param.Battery_Cell.Istar A  delta=HEV_Param.Battery_Cell.delta  Tau1=HEV_Param.Battery_Cell.Tau1 s  Qinit=HEV_Param.Battery_Cell.Qe_init s*A  i_Log=off  Iavg_Log=off  Qe_Log=off  LocalVarNames=|i|v|cap_u|cap_t|Q|Iavg  LocalVarDescs=|Current through variable|Voltage across variable|usable battery capacity|total battery capacity|battery charge|average current given by (I/(Ts+1))  LocalVarLogging=[0 0 0 0 0 0]
  R0 : LeadAcidBattery_lib/Terminal Resistance, R0  R00=HEV_Param.Battery_Cell.Roo Ohm  A0=HEV_Param.Battery_Cell.Ao  i_Log=off  LocalVarNames=|i|v  LocalVarDescs=|Current through variable|Voltage across variable  LocalVarLogging=[0 0]
  R1 : LeadAcidBattery_lib/Main Branch Resistance, R1  R10=HEV_Param.Battery_Cell.R10 Ohm  DOC_min=1e-006  i_Log=off  LocalVarNames=|i|v  LocalVarDescs=|Current through variable|Voltage across variable  LocalVarLogging=[0 0]
  R2 : LeadAcidBattery_lib/Main Branch Resistance, R2  R20=HEV_Param.Battery_Cell.R20 Ohm  A21=HEV_Param.Battery_Cell.A21  A22=HEV_Param.Battery_Cell.A22  Istar=HEV_Param.Battery_Cell.Istar A  i_Log=off  LocalVarNames=|i|v  LocalVarDescs=|Current through variable|Voltage across variable  LocalVarLogging=[0 0]
  Rp : LeadAcidBattery_lib/Parasitic Branch Resistance, Rp  Gp0=HEV_Param.Battery_Cell.Gpo 1/Ohm  Vp0=HEV_Param.Battery_Cell.Vpo V  Ap=HEV_Param.Battery_Cell.Ap  Tf=HEV_Param.Battery_Cell.theta_f C  i_Log=off  LocalVarNames=|i|v|Vavg  LocalVarDescs=|Current through variable|Voltage across variable|average voltage given by (V/(Ts+1))  LocalVarLogging=[0 0 0]
  Thermal Model : Subsystem
  H : PMIOPort  Tag=PMCPort  Port=1  Side=Left
  + : PMIOPort  Tag=PMCPort  Port=2  Side=Left
  - : PMIOPort  Tag=PMCPort  Port=3  Side=Right
  connections:
  Diode/LConn1 -- R0/RConn1 -- R2/LConn2
  R2/RConn2 -- Thermal Model/LConn1
  -/RConn1 -- Ep/RConn1 -- Main Branch Voltage Source (Em)/RConn1
  Thermal Model/RConn1 -- Main Branch Voltage Source (Em)/RConn3
  Diode/RConn1 -- Rp/LConn1
  Ep/LConn1 -- Rp/RConn2
  Thermal Model/LConn2 -- H/RConn1
  R0/LConn1 -- R2/LConn1 -- Main Branch Voltage Source (Em)/LConn1
  R1/LConn2 -- C1/LConn1
  R1/LConn1 -- C1/LConn2 -- R2/RConn1
  Main Branch Voltage Source (Em)/LConn3 -- C1/RConn1 -- R1/RConn2
  R1/RConn1 -- Main Branch Voltage Source (Em)/LConn2
  R0/LConn2 -- +/RConn1
  Thermal Model/RConn2 -- Main Branch Voltage Source (Em)/RConn2 -- Rp/RConn1
